simulink model "HIL_Lidar_Slam_Sim"  (R2023a)
settings: Solver=FixedStepAuto  StartTime=0.0  StopTime=inf  RelTol=1e-3
model workspace (MAT data in the model file):
  SL_ROS_VariableLengthArrays_MaxSizes.CommonInfo.ArrayTruncateAction = 'EmitWarning'
  SL_ROS_VariableLengthArrays_MaxSizes.MsgTypeMap = containers.Map
  SL_ROS_VariableLengthArrays_MaxSizes.MsgTypeMap.serialization.keys = {'sensor_msgs/LaserScan'}
  SL_ROS_VariableLengthArrays_MaxSizes.MsgTypeMap.serialization.values{1}(1).PropertyName = 'Intensities'
  SL_ROS_VariableLengthArrays_MaxSizes.MsgTypeMap.serialization.values{1}(1).DataType = 'single'
  SL_ROS_VariableLengthArrays_MaxSizes.MsgTypeMap.serialization.values{1}(1).MaxLength = 1081
  SL_ROS_VariableLengthArrays_MaxSizes.MsgTypeMap.serialization.values{1}(2).PropertyName = 'Ranges'
  SL_ROS_VariableLengthArrays_MaxSizes.MsgTypeMap.serialization.values{1}(2).DataType = 'single'
  SL_ROS_VariableLengthArrays_MaxSizes.MsgTypeMap.serialization.values{1}(2).MaxLength = 1081
  SL_ROS_VariableLengthArrays_MaxSizes.MsgTypeMap.serialization.uniformity = 0
  SL_ROS_VariableLengthArrays_MaxSizes.MsgTypeMap.serialization.keyType = 'char'
  SL_ROS_VariableLengthArrays_MaxSizes.MsgTypeMap.serialization.valueType = 'any'
values from neighbouring files (symbols this model uses):
  pose = poses(end,:)    [LidarSlam_interp.m]
  scan = lidarScan(ranges,angles)    [LidarSlam_interp.m]
  slamStatus = int8(1)    [LidarSlam_interp.m]
undefined symbols (not defined in the file or in its folder): Angular, gray, Linear, Theta, X, Y
libraries: robotlib x8, visiontextngfix x5, simulink x2, visionanalysis x1
settings Model: Creator=Ron  LastModifiedBy=이승신
settings OptimizationCC: EnhancedBackFolding=on  PassReuseOutputArgsAs=Individual arguments  ZeroExternalMemoryAtStartup=off  ZeroInternalMemoryAtStartup=off  MaxStackSize=64  OptimizeBlockOrder=speed  DifferentSizesBufferReuse=on  OptimizationCustomize=off  EfficientTunableParamExpr=on
settings DebuggingCC: ParameterTunabilityLossMsg=error  UnconnectedInputMsg=warning  UnconnectedOutputMsg=warning  UnconnectedLineMsg=warning
settings HardwareCC: ProdBitPerPointer=32  ProdBitPerSizeT=32  ProdBitPerPtrDiffT=32  ProdLargestAtomicFloat=None  ProdIntDivRoundTo=Undefined  ProdEndianess=Unspecified  ProdWordSize=32  ProdHWDeviceType=Generic->Unspecified (assume 32-bit Generic)
settings ModelReferenceCC: EnableRefExpFcnMdlSchedulingChecks=on
settings RTWCC: Description=Embedded Coder  SystemTargetFile=ert.tlc  HardwareBoard=Robot Operating System (ROS)  TLCOptions="-aInlineSetEventsForThisBaseRateFcn=TLC_FALSE -aSuppressMultiTaskScheduler=TLC_FALSE    -aRateBasedStepFcn=0"  TemplateMakefile=ert_default_tmf  Toolchain=Catkin  TargetLang=C++  CheckMdlBeforeBuild=Warning  DLArmComputeVersion=19.05
settings CodeAppCC: ForceParamTrailComments=on  IgnoreCustomStorageClasses=off  OperatorAnnotations=on  SimulinkDataObjDesc=on  SFDataObjDesc=on  InsertBlockDesc=on
settings ERTTargetCC: SupportNonInlinedSFcns=on  SupportVariableSizeSignals=on  ExtModeMexArgs='192.168.80.136' 0 17725  RootIOFormat=Structure reference

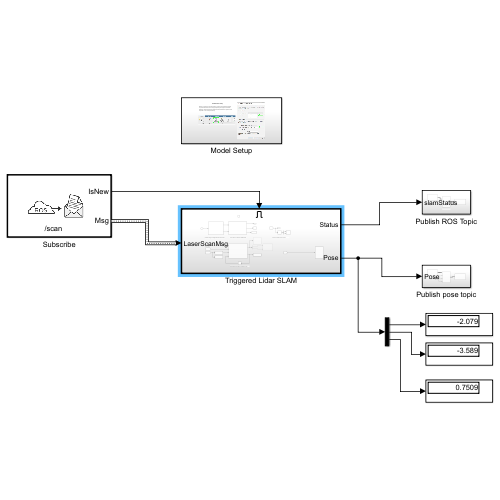
[thumbnail: Simulink's stored preview of the top-level diagram]
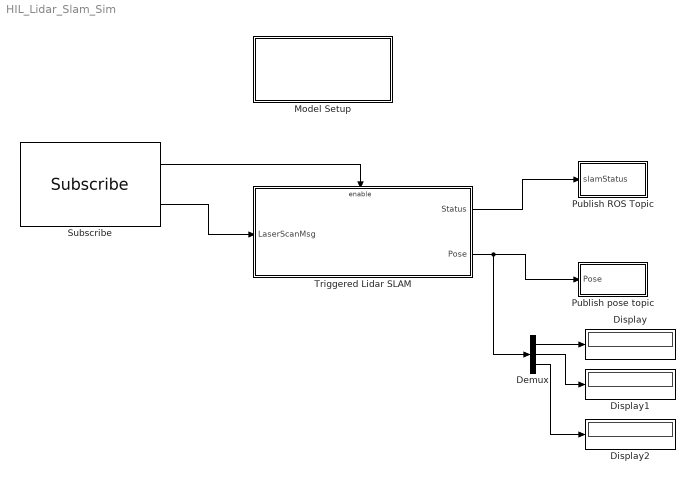
== system HIL_Lidar_Slam_Sim ==
  Demux : Demux  Outputs=3
  Display : Display
  Display1 : Display
  Display2 : Display
  Model Setup : Subsystem
  Publish ROS Topic : Subsystem
  Publish pose topic : Subsystem
  Subscribe : robotlib/Subscribe  topicSource=Select from ROS network  topic=/scan  messageType=sensor_msgs/LaserScan  SampleTime=-1  legacyBusStruct=off  messageQueueLength=1
  Triggered Lidar SLAM : Subsystem
  wires:
  Subscribe/1 -> Triggered Lidar SLAM/Enable
  Subscribe/2 -> Triggered Lidar SLAM/1(LaserScanMsg)
  Triggered Lidar SLAM/1(Status) -> Publish ROS Topic/1(slamStatus)
  Triggered Lidar SLAM/2(Pose) -> Demux/1, Publish pose topic/1(Pose)
  Demux/1 -> Display/1
  Demux/2 -> Display1/1
  Demux/3 -> Display2/1

== system HIL_Lidar_Slam_Sim/Model Setup ==
  note: Before running the Simulink model, make sure the ROS network requirements have been set appropriately through the Simulink Toolstrip. Note that setting a Node Host IP address is optional and depends on the computer setup.
  note: ROS Model Setup

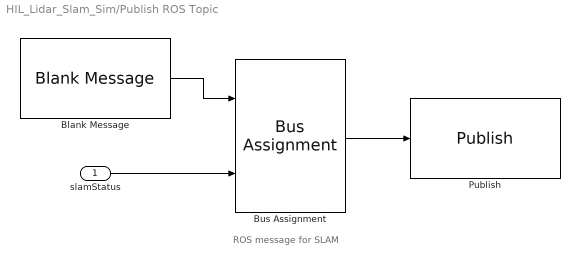
== system HIL_Lidar_Slam_Sim/Publish ROS Topic ==
  note: ROS message for SLAM
  slamStatus : Inport
  Blank Message : robotlib/Blank Message  messageClass=Message  entityType=std_msgs/Int8  messageType=std_msgs/Int8  SampleTime=inf  legacyBusStruct=off
  Bus Assignment : BusAssignment  AssignedSignals=Data
  Publish : robotlib/Publish  topicSource=Specify your own  topic=/slamStatus  messageType=std_msgs/Int8  legacyBusStruct=off  messageQueueLength=1
  wires:
  Bus Assignment/1 -> Publish/1
  Blank Message/1 -> Bus Assignment/1
  slamStatus/1 -> Bus Assignment/2

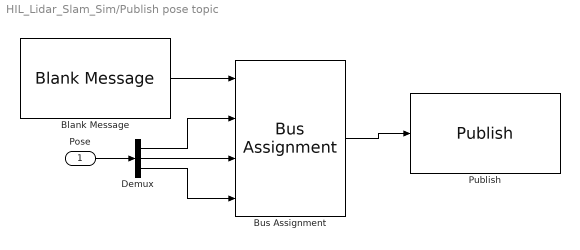
== system HIL_Lidar_Slam_Sim/Publish pose topic ==
  Pose : Inport
  Blank Message : robotlib/Blank Message  messageClass=Message  entityType=geometry_msgs/Pose2D  messageType=geometry_msgs/Pose2D  SampleTime=inf  legacyBusStruct=off
  Bus Assignment : BusAssignment  AssignedSignals=X,Y,Theta
  Demux : Demux  Outputs=3
  Publish : robotlib/Publish  topicSource=Specify your own  topic=/pose  messageType=geometry_msgs/Pose2D  legacyBusStruct=off  messageQueueLength=1
  wires:
  Blank Message/1 -> Bus Assignment/1
  Bus Assignment/1 -> Publish/1
  Pose/1 -> Demux/1
  Demux/3 -> Bus Assignment/4
  Demux/1 -> Bus Assignment/2
  Demux/2 -> Bus Assignment/3

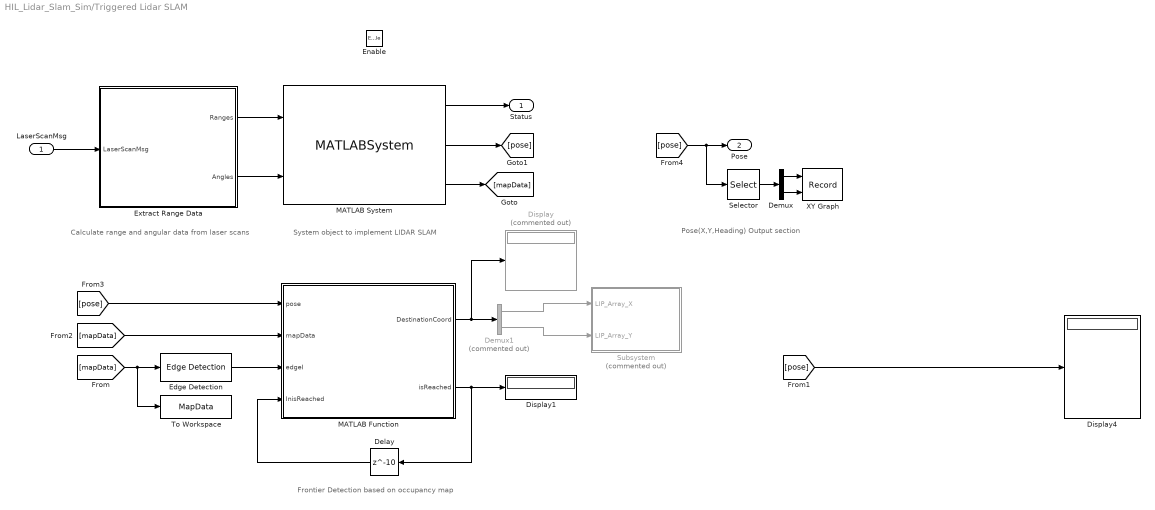
== system HIL_Lidar_Slam_Sim/Triggered Lidar SLAM ==
  note: Calculate range and angular data from laser scans
  note: System object to implement LIDAR SLAM
  note: Frontier Detection based on occupancy map
  note: Pose(X,Y,Heading) Output section
  LaserScanMsg : Inport
  Enable : EnablePort  PropagateVarSize=During execution
  Delay : Delay  DelayLength=10
  Demux : Demux  Outputs=2
  Demux1 : Demux  Commented=on  Outputs=2
  Display : Display  Commented=on
  Display1 : Display
  Display4 : Display
  Edge Detection : visionanalysis/Edge Detection  method=Sobel  outputType=Binary image  userDefinedThreshold=off  thresholdSource=Input port  threshold=20  thresholdTuning=4  edgeThinning=off  threshold_canny=[0.25 0.60]  autoPercent=70  sigma=1  roundingMode=Floor  overflowMode=off  prodOutputMode=Binary point scaling  prodOutputWordLength=32  prodOutputFracLength=8
  Extract Range Data : MATLAB Function  TreatAsAtomicUnit=on
  MATLAB Function : MATLAB Function  TreatAsAtomicUnit=on
  MATLAB System : MATLABSystem  System=LidarSlam_interp  maxLidarRange=10  mapResolution=20  maxNumScans=15  SimulateUsing=Interpreted execution
      mask Type: LidarSlam_interp
      mask Display:
      | disp('LidarSlam_interp');
      | port_label('input',1,'ranges');
      | port_label('input',2,'angles');
      | port_label('output',1,'slamStatus');
      | port_label('output',2,'pose');
      | port_label('output',3,'mapData');
  Selector : Selector  InputPortWidth=3  IndexOptions=Index vector (dialog)  Indices=[1 2]  OutputSizes=1
  Subsystem : Subsystem  Commented=on
  To Workspace : ToWorkspace  VariableName=MapData  SaveFormat=Structure With Time  SampleTime=-1
  XY Graph : Record  FileSettingsInternal="{\"entries\":[{\"content\":{\"excelSettings\":{\"content\":{},\"type\":\"Streamout.ExcelSettings\"}},\"type\":\"Streamout.FileSettingStorage\",\"uuid\":\"\"}],\"packageUris\":[\"http:\\/\\/schema.mathworks.com\\/mf0\\/streamout_blocks\\/R2020a\"],\"version\":\"1.0\"}"  Layout=[1 1]  SignalsInternal="{\"entries\":[{\"content\":{\"signals\":[{\"content\":{\"blockPath\":[],\"dimensions\":[1,1],\"domain\":\"\",\"lineColor\":\"#a2142f\",\"plots\":[1],\"port\":1,\"sid\":[\"\"],\"signalID\":932,\"signalName\":\"Demux:1\"},\"type\":\"RecordBlkView.Signal\",\"uuid\":\"\"},{\"content\":{\"blockPath\":[],\"dimensions\":[1,1],\"domain\":\"\",\"lineColor\":\"#139fff\",\"plots\":[1],\"port\":2,\"sid\":[\"\"],\"signalID\":936,\"signalName\":\"Demux:2\"},\"type\":\"RecordBlkView.Signal\",\"uuid\":\"\"}]},\"type\":\"RecordBlkView.InputSignals\",\"uuid\":\"\"}],\"packageUris\":[\"http:\\/\\/schema.mathworks.com\\/mf0\\/streamout_blocks\\/R2020a\"],\"version\":\"1.0\"}"  VisualizationBindings="{\"xyplotplugin\":{\"info\":[{\"series\":[{\"bindingParametersList\":[{\"parameter\":\"X-Axis\",\"signalID\":932,\"signalName\":\"Demux:1\"},{\"parameter\":\"Y-Axis\",\"signalID\":936,\"signalName\":\"Demux:2\"}],\"seriesID\":63206}],\"subplotID\":1}]}}"  CompatibilityTag=XY  st=-1
  Status : Outport
  Pose : Outport  Port=2
  wires:
  LaserScanMsg/1 -> Extract Range Data/1(LaserScanMsg)
  MATLAB System/1 -> Status/1
  Demux/2 -> XY Graph/2
  Demux/1 -> XY Graph/1
  Selector/1 -> Demux/1
  Extract Range Data/1(Ranges) -> MATLAB System/1
  Extract Range Data/2(Angles) -> MATLAB System/2
  Edge Detection/1 -> MATLAB Function/3(edgeI)
  MATLAB Function/1(DestinationCoord) -> Display/1, Demux1/1
  MATLAB Function/2(isReached) -> Delay/1, Display1/1
  Delay/1 -> MATLAB Function/4(InisReached)
  MATLAB System/2 -> [pose]
  MATLAB System/3 -> [mapData]
  [mapData] -> To Workspace/1, Edge Detection/1
  [mapData] -> MATLAB Function/2(mapData)
  [pose] -> MATLAB Function/1(pose)
  [pose] -> Selector/1, Pose/1
  Demux1/1 -> Subsystem/1(LIP_Array_X)
  Demux1/2 -> Subsystem/2(LIP_Array_Y)
  [pose] -> Display4/1

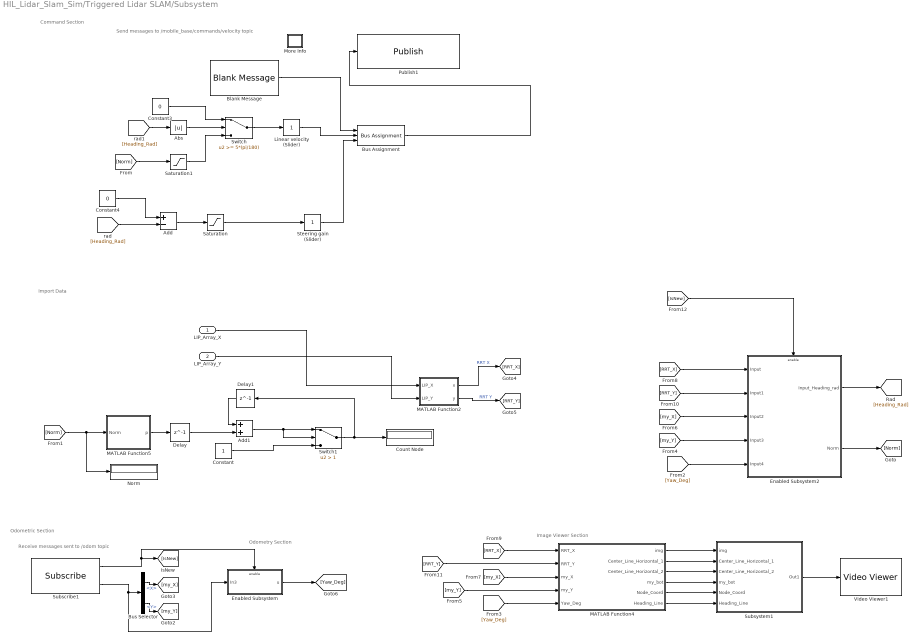
== system HIL_Lidar_Slam_Sim/Triggered Lidar SLAM/Subsystem ==
  note: Command Section
  note: Odometry Section
  note: Image Viewer Section
  note: Import Data
  note: Odometric Section
  note: Receive messages sent to /odom topic
  note: Send messages to /mobile_base/commands/velocity topic
  LIP_Array_X : Inport
  LIP_Array_Y : Inport  Port=2
  Abs : Abs  SaturateOnIntegerOverflow=off
  Add : Sum  Inputs=+-
  Add1 : Sum
  Blank Message : robotlib/Blank Message  messageClass=Message  entityType=geometry_msgs/Twist  messageType=geometry_msgs/Twist  SampleTime=0.01  legacyBusStruct=off
  Bus Assignment : BusAssignment  DialogController=Simulink.DDGSource_BusAssignment  AssignedSignals=Linear.X,Angular.Z
  Bus Selector : BusSelector  DialogController=Simulink.DDGSource_BusSelector  OutputSignals=Pose.Pose.Position.X,Pose.Pose.Position.Y
  Constant : Constant
  Constant3 : Constant  Value=0
  Constant4 : Constant  Value=0
  Count Node : Display
  Delay : Delay  DelayLength=1
  Delay1 : Delay  DelayLength=1
  Enabled Subsystem : Subsystem  TreatAsAtomicUnit=on
  Enabled Subsystem2 : Subsystem  TreatAsAtomicUnit=on
  Linear velocity (Slider) : simulink/Math Operations/Slider Gain  gain=1  low=0  high=2
  MATLAB Function2 : MATLAB Function  TreatAsAtomicUnit=on
  MATLAB Function4 : MATLAB Function  TreatAsAtomicUnit=on
  MATLAB Function5 : MATLAB Function  TreatAsAtomicUnit=on
  More Info : Subsystem
      settings: OpenFcn=showdemo(bdroot(gcb))
      mask Display: disp('?')
  Norm : Display
  Publish1 : robotlib/Publish  topicSource=Select from ROS network  topic=/cmd_vel  messageType=geometry_msgs/Twist  legacyBusStruct=off  messageQueueLength=105
  Saturation : Saturate  UpperLimit=0.3  LowerLimit=-0.3
  Saturation1 : Saturate  UpperLimit=0.3  LowerLimit=-0.3
  Steering gain (Slider) : simulink/Math Operations/Slider Gain  gain=1  low=-1  high=1
  Subscribe1 : robotlib/Subscribe  topicSource=Select from ROS network  topic=/odom  messageType=nav_msgs/Odometry  SampleTime=-1  legacyBusStruct=off  messageQueueLength=51
  Subsystem1 : Subsystem
  Switch : Switch  Threshold=5*(pi/180)  SaturateOnIntegerOverflow=off  InputSameDT=off
  Switch1 : Switch  Criteria=u2 > Threshold  Threshold=1  SaturateOnIntegerOverflow=off  InputSameDT=off
  Video Viewer1 : VideoViewer  colormapValue=gray(256)  FigPos=[755 1049 776 766]
  wires:
  Saturation/1 -> Steering gain (Slider)/1
  Subsystem1/1(Out1) -> Video Viewer1/1
  [Norm] -> Saturation1/1
  [Heading_Rad] -> Add/2
  Enabled Subsystem/1(u) -> [Yaw_Deg]
  Delay1/1 -> Add1/1
  MATLAB Function4/1(img) -> Subsystem1/1(img)
  [Yaw_Deg] -> MATLAB Function4/5(Yaw_Deg)
  Add/1 -> Saturation/1
  Steering gain (Slider)/1 -> Bus Assignment/3
  Switch/1 -> Linear velocity (Slider)/1
  Bus Assignment/1 -> Publish1/1
  MATLAB Function4/5(Node_Coord) -> Subsystem1/5(Node_Coord)
  [my_X] -> Enabled Subsystem2/3(Input2)
  Blank Message/1 -> Bus Assignment/1
  MATLAB Function4/4(my_bot) -> Subsystem1/4(my_bot)
  LIP_Array_X/1 -> MATLAB Function2/1(LIP_X)
  MATLAB Function4/3(Center_Line_Horizontal_2) -> Subsystem1/3(Center_Line_Horizontal_2)
  MATLAB Function5/1(p) -> Delay/1
  Add1/1 -> Switch1/1, Switch1/2
  [my_X] -> MATLAB Function4/3(my_X)
  [RRT_X] -> MATLAB Function4/1(RRT_X)
  Enabled Subsystem2/2(Norm) -> [Norm]
  [my_Y] -> MATLAB Function4/4(my_Y)
  [Norm] -> Norm/1, MATLAB Function5/1(Norm)
  MATLAB Function2/2(y) -> [RRT_Y]  "RRT Y"
  Enabled Subsystem2/1(Input_Heading_rad) -> [Heading_Rad]
  Delay/1 -> Add1/2
  [IsNew] -> Enabled Subsystem2/Enable
  Saturation1/1 -> Switch/3
  Constant/1 -> Switch1/3
  MATLAB Function4/6(Heading_Line) -> Subsystem1/6(Heading_Line)
  [Yaw_Deg] -> Enabled Subsystem2/5(Input4)
  LIP_Array_Y/1 -> MATLAB Function2/2(LIP_Y)
  MATLAB Function2/1(x) -> [RRT_X]  "RRT X"
  Switch1/1 -> Count Node/1, Delay1/1
  Linear velocity (Slider)/1 -> Bus Assignment/2
  [RRT_X] -> Enabled Subsystem2/1(Input)
  [Heading_Rad] -> Abs/1
  Constant4/1 -> Add/1
  Abs/1 -> Switch/2
  [my_Y] -> Enabled Subsystem2/4(Input3)
  Constant3/1 -> Switch/1
  [RRT_Y] -> Enabled Subsystem2/2(Input1)
  MATLAB Function4/2(Center_Line_Horizontal_1) -> Subsystem1/2(Center_Line_Horizontal_1)
  [RRT_Y] -> MATLAB Function4/2(RRT_Y)
  Subscribe1/2 -> Bus Selector/1, Enabled Subsystem/1(In3)
  Subscribe1/1 -> Enabled Subsystem/Enable, [IsNew]
  Bus Selector/1 -> [my_X]  "<X>"
  Bus Selector/2 -> [my_Y]  "<Y>"

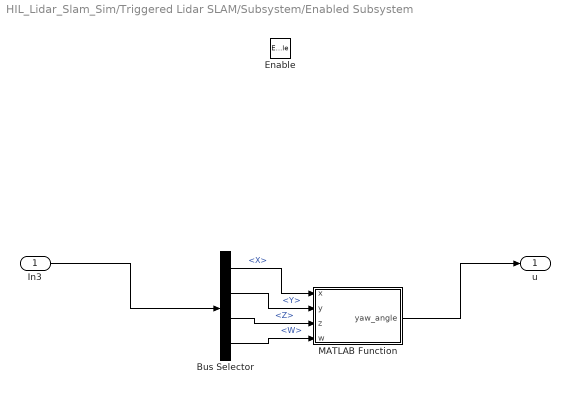
== system HIL_Lidar_Slam_Sim/Triggered Lidar SLAM/Subsystem/Enabled Subsystem ==
  In3 : Inport
  Enable : EnablePort
  Bus Selector : BusSelector  OutputSignals=Pose.Pose.Orientation.X,Pose.Pose.Orientation.Y,Pose.Pose.Orientation.Z,Pose.Pose.Orientation.W
  MATLAB Function : MATLAB Function  TreatAsAtomicUnit=on
  u : Outport
  wires:
  In3/1 -> Bus Selector/1
  Bus Selector/1 -> MATLAB Function/1(x)  "<X>"
  Bus Selector/2 -> MATLAB Function/2(y)  "<Y>"
  Bus Selector/3 -> MATLAB Function/3(z)  "<Z>"
  Bus Selector/4 -> MATLAB Function/4(w)  "<W>"
  MATLAB Function/1(yaw_angle) -> u/1

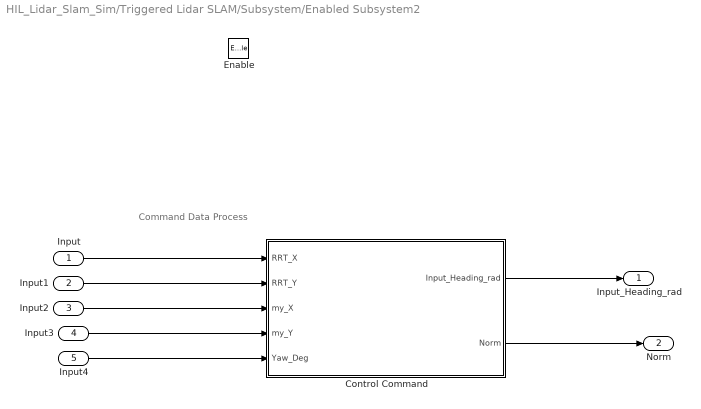
== system HIL_Lidar_Slam_Sim/Triggered Lidar SLAM/Subsystem/Enabled Subsystem2 ==
  note: Command Data Process
  Input : Inport
  Input1 : Inport  Port=2
  Input2 : Inport  Port=3
  Input3 : Inport  Port=4
  Input4 : Inport  Port=5
  Enable : EnablePort
  Control Command : MATLAB Function  TreatAsAtomicUnit=on
  Input_Heading_rad : Outport
  Norm : Outport  Port=2
  wires:
  Control Command/1(Input_Heading_rad) -> Input_Heading_rad/1
  Input4/1 -> Control Command/5(Yaw_Deg)
  Input2/1 -> Control Command/3(my_X)
  Control Command/2(Norm) -> Norm/1
  Input/1 -> Control Command/1(RRT_X)
  Input3/1 -> Control Command/4(my_Y)
  Input1/1 -> Control Command/2(RRT_Y)

== system HIL_Lidar_Slam_Sim/Triggered Lidar SLAM/Subsystem/More Info ==

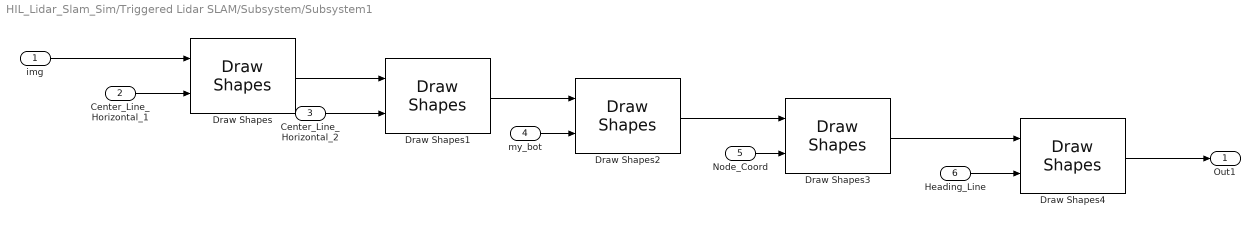
== system HIL_Lidar_Slam_Sim/Triggered Lidar SLAM/Subsystem/Subsystem1 ==
  img : Inport
  Center_Line_Horizontal_1 : Inport  Port=2
  Center_Line_Horizontal_2 : Inport  Port=3
  my_bot : Inport  Port=4
  Node_Coord : Inport  Port=5
  Heading_Line : Inport  Port=6
  Draw Shapes : visiontextngfix/Draw Shapes  shape=Lines  fill=off  lineWidth=1  fillClrSource=Specify via dialog  display=Black  intensity=200  color=[255 0 0]  opacity=0.6  viewport=Entire image  antialiasing=off  inType=Obsolete  imagePorts=One multidimensional signal  roundingMode=Floor  overflowMode=off  memoryMode=Specify word length  memoryWordLength=16  prodOutputMode=Binary point scaling  prodOutputWordLength=32  prodOutputFracLength=14  memoryFracLength=15
  Draw Shapes1 : visiontextngfix/Draw Shapes  shape=Lines  fill=off  lineWidth=1  fillClrSource=Specify via dialog  display=Black  intensity=200  color=[200 255 100]  opacity=0.6  viewport=Entire image  antialiasing=off  inType=Obsolete  imagePorts=One multidimensional signal  roundingMode=Floor  overflowMode=off  memoryMode=Specify word length  memoryWordLength=16  prodOutputMode=Binary point scaling  prodOutputWordLength=32  prodOutputFracLength=14  memoryFracLength=15
  Draw Shapes2 : visiontextngfix/Draw Shapes  shape=Circles  fill=off  lineWidth=3  fillClrSource=Specify via dialog  display=Black  intensity=200  color=[200 255 100]  opacity=0.6  viewport=Entire image  antialiasing=off  inType=Obsolete  imagePorts=One multidimensional signal  roundingMode=Floor  overflowMode=off  memoryMode=Specify word length  memoryWordLength=16  prodOutputMode=Binary point scaling  prodOutputWordLength=32  prodOutputFracLength=14  memoryFracLength=15
  Draw Shapes3 : visiontextngfix/Draw Shapes  shape=Circles  fill=on  lineWidth=1  fillClrSource=Specify via dialog  display=Black  intensity=200  color=[200 255 100]  opacity=0.6  viewport=Entire image  antialiasing=off  inType=Obsolete  imagePorts=One multidimensional signal  roundingMode=Floor  overflowMode=off  memoryMode=Specify word length  memoryWordLength=16  prodOutputMode=Binary point scaling  prodOutputWordLength=32  prodOutputFracLength=14  memoryFracLength=15
  Draw Shapes4 : visiontextngfix/Draw Shapes  shape=Lines  fill=off  lineWidth=1  fillClrSource=Specify via dialog  display=Black  intensity=200  color=[200 255 100]  opacity=0.6  viewport=Entire image  antialiasing=off  inType=Obsolete  imagePorts=One multidimensional signal  roundingMode=Floor  overflowMode=off  memoryMode=Specify word length  memoryWordLength=16  prodOutputMode=Binary point scaling  prodOutputWordLength=32  prodOutputFracLength=14  memoryFracLength=15
  Out1 : Outport
  wires:
  Draw Shapes1/1 -> Draw Shapes2/1
  Node_Coord/1 -> Draw Shapes3/2
  Draw Shapes/1 -> Draw Shapes1/1
  Draw Shapes2/1 -> Draw Shapes3/1
  Draw Shapes3/1 -> Draw Shapes4/1
  Center_Line_Horizontal_2/1 -> Draw Shapes1/2
  Center_Line_Horizontal_1/1 -> Draw Shapes/2
  my_bot/1 -> Draw Shapes2/2
  img/1 -> Draw Shapes/1
  Heading_Line/1 -> Draw Shapes4/2
  Draw Shapes4/1 -> Out1/1

== matlab function HIL_Lidar_Slam_Sim/Triggered Lidar SLAM/MATLAB Function ==
  data: pose input; DestinationCoord output; mapData input; edgeI input; isReached output; InisReached input
function [DestinationCoord, isReached]  = FrontierDetection(pose,mapData,edgeI,InisReached)
persistent goalCoordinate
if(isempty(goalCoordinate))
    goalCoordinate = [0 0];
end

if(~isempty(mapData))
    [row , ~] = find(isnan(mapData));

    if(~isempty(row))
        mapData = mapData(1:row(1)-1,1:row(1)-1);
    else
        mapData = mapData;
    end
    map = occupancyMap(mapData,20);
    map.GridOriginInLocal = [-10 -10];

    %% Frontier Detection
    sobel = edgeI;
    [idx_x,idx_y] = find(sobel == 1);
    edgeCoord = [idx_x, idx_y];
    frontier = [];

    for ii = 1:length(edgeCoord)
        % WARNING WARNIGN
        % xl, xr ... 계산하는데 인덱스 초과 예외코드 없음. 향후 오류 발생 가능성 존재
        x = edgeCoord(ii,1); y = edgeCoord(ii,2);
        xl = x-1; yl = y;
        xr = x+1; yr = y;
        xu = x; yu = y-1;
        xd = x; yd = y+1;
        if(mapData(x,y) > 0.1)
            continue
        end

        if(mapData(xl,yl) > 0.49 && mapData(xl,yl) < 0.51) % Unknown area
            cord = grid2world(map,[x,y]);
            frontier = [frontier; cord(1),cord(2)];

        elseif(mapData(xr,yr) > 0.49 && mapData(xr,yr) < 0.51)
            cord = grid2world(map,[x,y]);
            frontier = [frontier; cord(1),cord(2)];

        elseif(mapData(xu,yu) > 0.49 && mapData(xu,yu) < 0.51)
            cord = grid2world(map,[x,y]);
            frontier = [frontier; cord(1),cord(2)];

        elseif(mapData(xd,yd) > 0.49 && mapData(xd,yd) < 0.51)
            cord = grid2world(map,[x,y]);
            frontier = [frontier; cord(1),cord(2)];

        end
    end
    %% Set Goal Point
    randIdx = randi([1,length(frontier)],1,1);
    
    %% 목적지에 도달하면 -> 목적지와 거리가 goalDistance 이내라면
    goalDistance = 1;
    if(sqrt((pose(1)-goalCoordinate(1))^2 + (pose(2)-goalCoordinate(2))^2) < goalDistance && InisReached == 1)
        DestinationCoord = frontier(randIdx,:);
        scatter(DestinationCoord(1),DestinationCoord(2),'x','CData',[1 0 0]);
        goalCoordinate = DestinationCoord;
        isReached = 0;
    elseif(sqrt((pose(1)-goalCoordinate(1))^2 + (pose(2)-goalCoordinate(2))^2) < goalDistance && InisReached == 0)
        DestinationCoord = goalCoordinate;
        scatter(DestinationCoord(1),DestinationCoord(2),'x','CData',[1 0 0]);
        isReached = 1;
    else
        DestinationCoord = goalCoordinate;
        scatter(DestinationCoord(1),DestinationCoord(2),'x','CData',[1 0 0]);
        isReached = 0;
    end
    
    
    % Edge 검출 디버깅용, 검출된 Edge를 plotting 함
    %scatter(frontier(:,1), frontier(:,2),'x')

else
    DestinationCoord = [0 0];
    isReached = 0;
end

== matlab function HIL_Lidar_Slam_Sim/Triggered Lidar SLAM/Subsystem/Enabled Subsystem/MATLAB Function ==
  data: x input; yaw_angle output; y input; z input; w input
function yaw_angle  = fcn(x, y, z, w)

quat = [w x y z];
eul_angle = quat2eul(quat);
yaw_angle = rad2deg(eul_angle(1));

== matlab function HIL_Lidar_Slam_Sim/Triggered Lidar SLAM/Subsystem/Enabled Subsystem2/Control Command ==
  data: RRT_X input; RRT_Y input; my_X input; my_Y input; Yaw_Deg input; Input_Heading_rad output; Norm output
function [Input_Heading_rad,Norm]  = fcn(RRT_X, RRT_Y, my_X, my_Y, Yaw_Deg)

Vector = zeros(1,2);

Vector(1,1) = RRT_X - my_X;
Vector(1,2) = RRT_Y - my_Y;

Norm = norm(Vector);

Com_Vector = complex(Vector(1,1), Vector(1,2));

Heading_Rad = angle(Com_Vector);

Heading_Deg = rad2deg(Heading_Rad);

Ref_Heading = Yaw_Deg - Heading_Deg;

Input_Heading = 0;

if Ref_Heading > 180
    Input_Heading = Ref_Heading - 360;
elseif Ref_Heading < -180
    Input_Heading = 360 - Ref_Heading;
else
    Input_Heading = Ref_Heading;
end

Input_Heading_rad = (2*pi/360)*Input_Heading;


% coder.extrinsic('polarplot');
% 
% X = [my_X RRT_X];
% Y = [my_Y RRT_Y];
% 
% color = [1 7];
% 
% figure(2)
% scatter(X,Y,25,color,'filled');
% axis([-10 10 -10 10])

== matlab function HIL_Lidar_Slam_Sim/Triggered Lidar SLAM/Subsystem/MATLAB Function2 ==
  data: x output; LIP_X input; LIP_Y input; y output
function [x,y] = fcn(LIP_X, LIP_Y)

x = LIP_X(1,1);
y = LIP_Y(1,1);

== matlab function HIL_Lidar_Slam_Sim/Triggered Lidar SLAM/Extract Range Data ==
  data: LaserScanMsg input; Ranges output; Angles output
function [Ranges, Angles] = ExtractRangeData(LaserScanMsg)
%#codegen

% Extract Range information
Ranges = double(LaserScanMsg.Ranges);

% Construct Angles vector using AngleMin and AngleIncrement from sensor
% reading.
angMin = double(LaserScanMsg.AngleMin);
angIncrement = double(LaserScanMsg.AngleIncrement);

numReadings = numel(Ranges);
rawAngles = angMin + (0:numReadings-1)' * angIncrement;

% Wrap the angles to the (-pi,pi] interval.
Angles = robotics.internal.wrapToPi(double(rawAngles));

== matlab function HIL_Lidar_Slam_Sim/Triggered Lidar SLAM/Subsystem/MATLAB Function4 ==
  data: RRT_X input; img output; RRT_Y input; my_X input; my_Y input; Center_Line_Horizontal_1 output; Center_Line_Horizontal_2 output; my_bot output; Node_Coord output; Yaw_Deg input; Heading_Line output
function [img,Center_Line_Horizontal_1,Center_Line_Horizontal_2,my_bot,Node_Coord,Heading_Line] = fcn(RRT_X, RRT_Y, my_X, my_Y, Yaw_Deg)

img = ones(2048);

center = 2048/2;

Center_Line_Horizontal_1 = [center 1 center 2048];
Center_Line_Horizontal_2 = [1 center 2048 center];

my_col = center - my_Y;
my_row = center + my_X;

Node_col = center - RRT_Y;
Node_row = center + RRT_X;

my_bot = [my_row ,my_col,3; my_row,my_col,1];
Node_Coord = [Node_row, Node_col, 5; Node_row, Node_col, 2];

Yaw_Rad = deg2rad(Yaw_Deg);

Heading_Angle_X = my_X + 10*cos(Yaw_Rad);
Heading_Angle_Y = my_Y + 10*sin(Yaw_Rad);

Heading_col = center - Heading_Angle_Y;
Heading_row = center + Heading_Angle_X;

Heading_Line = [my_row my_col Heading_row Heading_col];

== matlab function HIL_Lidar_Slam_Sim/Triggered Lidar SLAM/Subsystem/MATLAB Function5 ==
  data: p output; Norm input
function p = fcn(Norm)
p = 0;

if Norm < 0.5
    p = 1;
end
